simulink model "InterlockDeadtime3L"  (R2025b)
settings: Solver=FixedStepDiscrete  StartTime=0.0  StopTime=0.0000004  RelTol=1e-3
undefined symbols (not defined in the file): T_FPGA_clk
libraries: simulink x3, hdlsllib x3
settings Model: PacingRate=0.010000  Creator=info  LastModifiedBy=info
settings OptimizationCC: BlockReduction=off  ConditionallyExecuteInputs=off  DefaultParameterBehavior=Inlined
settings DebuggingCC: AlgebraicLoopMsg=error
settings HardwareCC: ProdBitPerPointer=32.0  ProdBitPerSizeT=32.0  ProdBitPerPtrDiffT=32.0  ProdLargestAtomicFloat=None  ProdIntDivRoundTo=Undefined  ProdEndianess=Unspecified  ProdWordSize=32.0  ProdHWDeviceType=ASIC/FPGA->ASIC/FPGA  TargetBitPerPointer=64.0  TargetBitPerSizeT=64.0  TargetBitPerPtrDiffT=64.0  TargetLongLongMode=on  TargetIntDivRoundTo=Zero  TargetEndianess=LittleEndian  TargetWordSize=64.0  TargetHWDeviceType=Custom Processor->MATLAB Host Computer  ProdEqTarget=off

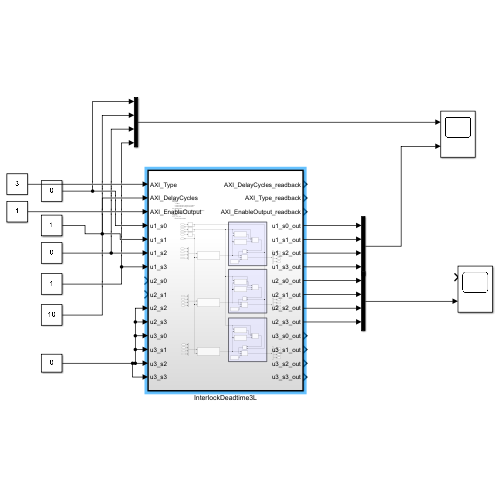
[thumbnail: Simulink's stored preview of the top-level diagram]
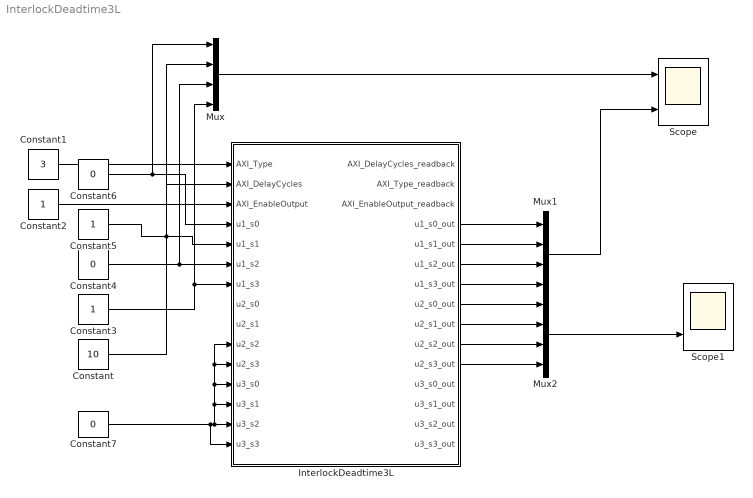
== system InterlockDeadtime3L ==
  Constant : Constant  Value=10  OutDataTypeStr=uint32  SampleTime=T_FPGA_clk
  Constant1 : Constant  Value=3  OutDataTypeStr=uint8  SampleTime=T_FPGA_clk
  Constant2 : Constant  OutDataTypeStr=boolean  SampleTime=T_FPGA_clk
  Constant3 : Constant  OutDataTypeStr=boolean  SampleTime=T_FPGA_clk
  Constant4 : Constant  Value=0  OutDataTypeStr=boolean  SampleTime=T_FPGA_clk
  Constant5 : Constant  OutDataTypeStr=boolean  SampleTime=T_FPGA_clk
  Constant6 : Constant  Value=0  OutDataTypeStr=boolean  SampleTime=T_FPGA_clk
  Constant7 : Constant  Value=0  OutDataTypeStr=boolean  SampleTime=T_FPGA_clk
  InterlockDeadtime3L : Subsystem  TreatAsAtomicUnit=on
  Mux : Mux
  Mux1 : Mux
  Mux2 : Mux
  Scope : Scope  NumInputPorts=2
      settings: ActiveDisplayYMinimum=-0.12499999999999997  ActiveDisplayYMaximum=1.125  DataLoggingVariableName=ScopeData2  DataLoggingSaveFormat=Array
  Scope1 : Scope  NumInputPorts=2
      settings: ActiveDisplayYMinimum=-0.12499999999999997  ActiveDisplayYMaximum=1.125  DataLoggingSaveFormat=Array
  wires:
  Constant/1 -> InterlockDeadtime3L/2(AXI_DelayCycles)
  Constant1/1 -> InterlockDeadtime3L/1(AXI_Type)
  Constant2/1 -> InterlockDeadtime3L/3(AXI_EnableOutput)
  Constant3/1 -> Mux/4, InterlockDeadtime3L/7(u1_s3)
  Constant6/1 -> Mux/1, InterlockDeadtime3L/4(u1_s0)
  Constant5/1 -> Mux/2, InterlockDeadtime3L/5(u1_s1)
  Constant4/1 -> Mux/3, InterlockDeadtime3L/6(u1_s2)
  Mux/1 -> Scope/1
  InterlockDeadtime3L/4(u1_s0_out) -> Mux1/1
  InterlockDeadtime3L/5(u1_s1_out) -> Mux1/2
  InterlockDeadtime3L/6(u1_s2_out) -> Mux1/3
  InterlockDeadtime3L/7(u1_s3_out) -> Mux1/4
  Mux1/1 -> Scope/2
  Constant7/1 -> InterlockDeadtime3L/15(u3_s3), InterlockDeadtime3L/14(u3_s2), InterlockDeadtime3L/13(u3_s1), InterlockDeadtime3L/12(u3_s0), InterlockDeadtime3L/11(u2_s3), InterlockDeadtime3L/10(u2_s2)
  InterlockDeadtime3L/8(u2_s0_out) -> Mux2/1
  InterlockDeadtime3L/10(u2_s2_out) -> Mux2/3
  InterlockDeadtime3L/9(u2_s1_out) -> Mux2/2
  InterlockDeadtime3L/11(u2_s3_out) -> Mux2/4
  Mux2/1 -> Scope1/2

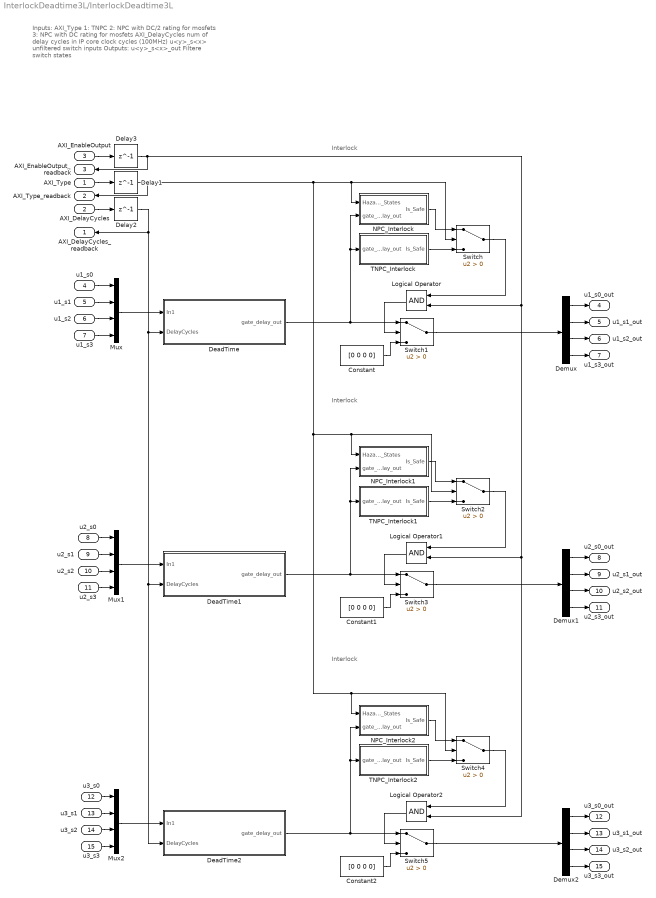
== system InterlockDeadtime3L/InterlockDeadtime3L ==
  note: Interlock
  note: Inputs:
      | AXI_Type
      | 1: TNPC
      | 2: NPC with DC/2 rating for mosfets
      | 3: NPC with DC rating for mosfets
      | AXI_DelayCycles
      | num of delay cycles in IP core clock cycles (100MHz)
      | u<y>_s<x>
      | unfiltered switch inputs
      | Outputs:
      | u<y>_s<x>_out
      | Filtere switch states
  note: Interlock
  note: Interlock
  AXI_Type : Inport
  AXI_DelayCycles : Inport  Port=2
  AXI_EnableOutput : Inport  Port=3
  u1_s0 : Inport  Port=4
  u1_s1 : Inport  Port=5
  u1_s2 : Inport  Port=6
  u1_s3 : Inport  Port=7
  u2_s0 : Inport  Port=8
  u2_s1 : Inport  Port=9
  u2_s2 : Inport  Port=10
  u2_s3 : Inport  Port=11
  u3_s0 : Inport  Port=12
  u3_s1 : Inport  Port=13
  u3_s2 : Inport  Port=14
  u3_s3 : Inport  Port=15
  Constant : Constant  Value=[0 0 0 0]  OutDataTypeStr=boolean
  Constant1 : Constant  Value=[0 0 0 0]  OutDataTypeStr=boolean
  Constant2 : Constant  Value=[0 0 0 0]  OutDataTypeStr=boolean
  DeadTime : Subsystem
  DeadTime1 : Subsystem
  DeadTime2 : Subsystem
  Delay1 : Delay  DelayLength=1
  Delay2 : Delay  DelayLength=1
  Delay3 : Delay  DelayLength=1
  Demux : Demux
  Demux1 : Demux
  Demux2 : Demux
  Logical Operator : Logic  AllPortsSameDT=off  OutDataTypeStr=boolean
  Logical Operator1 : Logic  AllPortsSameDT=off  OutDataTypeStr=boolean
  Logical Operator2 : Logic  AllPortsSameDT=off  OutDataTypeStr=boolean
  Mux : Mux
  Mux1 : Mux
  Mux2 : Mux
  NPC_Interlock : Subsystem
  NPC_Interlock1 : Subsystem
  NPC_Interlock2 : Subsystem
  Switch{,1..5} (6 alike) : Switch  Criteria=u2 > Threshold  SaturateOnIntegerOverflow=off  InputSameDT=off
  TNPC_Interlock : Subsystem
  TNPC_Interlock1 : Subsystem
  TNPC_Interlock2 : Subsystem
  AXI_DelayCycles_readback : Outport
  AXI_Type_readback : Outport  Port=2
  AXI_EnableOutput_readback : Outport  Port=3
  u1_s0_out : Outport  Port=4  OutDataTypeStr=boolean  VectorParamsAs1DForOutWhenUnconnected=off
  u1_s1_out : Outport  Port=5  OutDataTypeStr=boolean  VectorParamsAs1DForOutWhenUnconnected=off
  u1_s2_out : Outport  Port=6  OutDataTypeStr=boolean  VectorParamsAs1DForOutWhenUnconnected=off
  u1_s3_out : Outport  Port=7  OutDataTypeStr=boolean  VectorParamsAs1DForOutWhenUnconnected=off
  u2_s0_out : Outport  Port=8  OutDataTypeStr=boolean  VectorParamsAs1DForOutWhenUnconnected=off
  u2_s1_out : Outport  Port=9  OutDataTypeStr=boolean  VectorParamsAs1DForOutWhenUnconnected=off
  u2_s2_out : Outport  Port=10  OutDataTypeStr=boolean  VectorParamsAs1DForOutWhenUnconnected=off
  u2_s3_out : Outport  Port=11  OutDataTypeStr=boolean  VectorParamsAs1DForOutWhenUnconnected=off
  u3_s0_out : Outport  Port=12  OutDataTypeStr=boolean  VectorParamsAs1DForOutWhenUnconnected=off
  u3_s1_out : Outport  Port=13  OutDataTypeStr=boolean  VectorParamsAs1DForOutWhenUnconnected=off
  u3_s2_out : Outport  Port=14  OutDataTypeStr=boolean  VectorParamsAs1DForOutWhenUnconnected=off
  u3_s3_out : Outport  Port=15  OutDataTypeStr=boolean  VectorParamsAs1DForOutWhenUnconnected=off
  wires:
  u1_s0/1 -> Mux/1
  u1_s1/1 -> Mux/2
  u1_s2/1 -> Mux/3
  u1_s3/1 -> Mux/4
  Mux/1 -> DeadTime/1(In1)
  DeadTime/1(gate_delay_out) -> Switch1/1, NPC_Interlock/2(gate_delay_out), TNPC_Interlock/1(gate_delay_out)
  Demux/3 -> u1_s2_out/1
  Demux/4 -> u1_s3_out/1
  Demux/1 -> u1_s0_out/1
  Demux/2 -> u1_s1_out/1
  AXI_DelayCycles/1 -> Delay2/1
  AXI_Type/1 -> Delay1/1
  NPC_Interlock/1(Is_Safe) -> Switch/1
  TNPC_Interlock/1(Is_Safe) -> Switch/3
  Constant/1 -> Switch1/3
  Switch1/1 -> Demux/1
  Logical Operator/1 -> Switch1/2
  Switch/1 -> Logical Operator/1
  AXI_EnableOutput/1 -> Delay3/1
  Delay2/1 -> AXI_DelayCycles_readback/1, DeadTime2/2(DelayCycles), DeadTime1/2(DelayCycles), DeadTime/2(DelayCycles)
  Constant1/1 -> Switch3/3
  Switch3/1 -> Demux1/1
  Delay1/1 -> NPC_Interlock1/1(Hazard_States), Switch2/2, NPC_Interlock2/1(Hazard_States), Switch4/2, NPC_Interlock/1(Hazard_States), Switch/2, AXI_Type_readback/1
  TNPC_Interlock1/1(Is_Safe) -> Switch2/3
  Logical Operator1/1 -> Switch3/2
  NPC_Interlock1/1(Is_Safe) -> Switch2/1
  Switch2/1 -> Logical Operator1/1
  DeadTime1/1(gate_delay_out) -> Switch3/1, NPC_Interlock1/2(gate_delay_out), TNPC_Interlock1/1(gate_delay_out)
  Delay3/1 -> Logical Operator2/2, Logical Operator1/2, Logical Operator/2, AXI_EnableOutput_readback/1
  Constant2/1 -> Switch5/3
  Switch5/1 -> Demux2/1
  TNPC_Interlock2/1(Is_Safe) -> Switch4/3
  Logical Operator2/1 -> Switch5/2
  NPC_Interlock2/1(Is_Safe) -> Switch4/1
  Switch4/1 -> Logical Operator2/1
  DeadTime2/1(gate_delay_out) -> Switch5/1, NPC_Interlock2/2(gate_delay_out), TNPC_Interlock2/1(gate_delay_out)
  u2_s0/1 -> Mux1/1
  u2_s1/1 -> Mux1/2
  u2_s3/1 -> Mux1/4
  u2_s2/1 -> Mux1/3
  Mux1/1 -> DeadTime1/1(In1)
  u3_s0/1 -> Mux2/1
  u3_s1/1 -> Mux2/2
  u3_s2/1 -> Mux2/3
  u3_s3/1 -> Mux2/4
  Mux2/1 -> DeadTime2/1(In1)
  Demux1/4 -> u2_s3_out/1
  Demux1/1 -> u2_s0_out/1
  Demux1/2 -> u2_s1_out/1
  Demux1/3 -> u2_s2_out/1
  Demux2/4 -> u3_s3_out/1
  Demux2/1 -> u3_s0_out/1
  Demux2/2 -> u3_s1_out/1
  Demux2/3 -> u3_s2_out/1

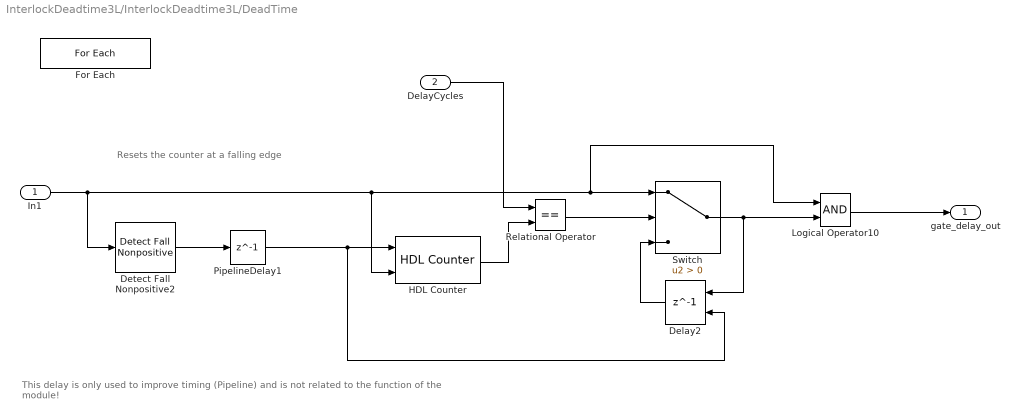
== system InterlockDeadtime3L/InterlockDeadtime3L/DeadTime ==
  note: This delay is only used to improve timing (Pipeline) and is not related to the function of the module!
  note: Resets the counter at a falling edge
  In1 : Inport  Partition=on  PartitionDimension=1  PartitionWidth=1  PartitionOffset=0
  DelayCycles : Inport  Port=2
  Delay2 : Delay  DelayLength=1  ExternalReset=Level  UseCircularBuffer=on
      settings: InputPortMap=u0,r5
  Detect Fall Nonpositive2 : simulink/Logic and Bit Operations/Detect Fall Nonpositive  vinit=0  OutDataTypeStr=boolean
  For Each : ForEach  DisableCoverage=on
  HDL Counter : hdlsllib/Sources/HDL Counter  CountType=Free running  CountInit=0  CountStep=1  CountMax=25  CountFromType=Initial value  CountFrom=0  CountResetPort=on  CountLoadPort=off  CountEnbPort=on  CountDirPort=off  CountHitOutputPort=off  CountDataType=Unsigned  CountWordLen=32  CountFracLen=0  CountSampTime=-1
  Logical Operator10 : Logic  AllPortsSameDT=off  OutDataTypeStr=boolean
  PipelineDelay1 : Delay  DelayLength=1
  Relational Operator : RelationalOperator  Operator===  OutDataTypeStr=boolean  RndMeth=Simplest  InputSameDT=off
  Switch : Switch  Criteria=u2 > Threshold  SaturateOnIntegerOverflow=off  InputSameDT=off
  gate_delay_out : Outport  ConcatenationDimension=1
  wires:
  Logical Operator10/1 -> gate_delay_out/1
  In1/1 -> Logical Operator10/1, Switch/1, HDL Counter/2, Detect Fall Nonpositive2/1
  HDL Counter/1 -> Relational Operator/2
  Delay2/1 -> Switch/3
  DelayCycles/1 -> Relational Operator/1
  Relational Operator/1 -> Switch/2
  PipelineDelay1/1 -> HDL Counter/1, Delay2/2
  Detect Fall Nonpositive2/1 -> PipelineDelay1/1
  Switch/1 -> Delay2/1, Logical Operator10/2

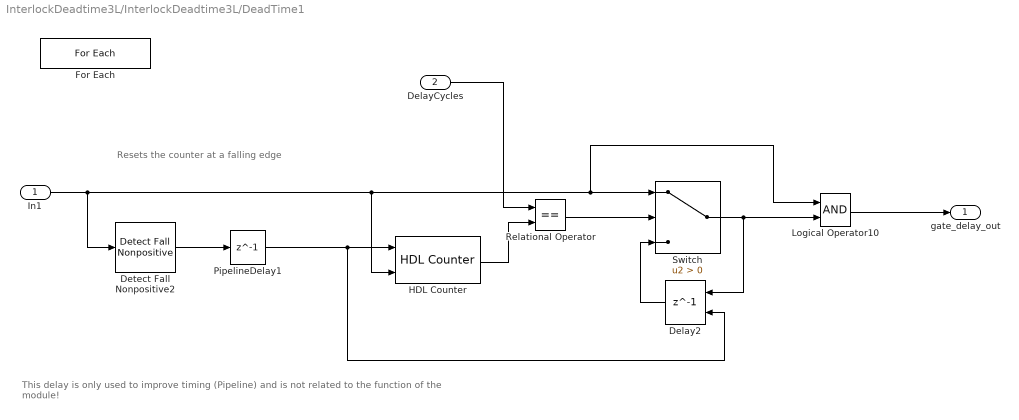
== system InterlockDeadtime3L/InterlockDeadtime3L/DeadTime1 ==
  note: This delay is only used to improve timing (Pipeline) and is not related to the function of the module!
  note: Resets the counter at a falling edge
  In1 : Inport  Partition=on  PartitionDimension=1  PartitionWidth=1  PartitionOffset=0
  DelayCycles : Inport  Port=2
  Delay2 : Delay  DelayLength=1  ExternalReset=Level  UseCircularBuffer=on
      settings: InputPortMap=u0,r5
  Detect Fall Nonpositive2 : simulink/Logic and Bit Operations/Detect Fall Nonpositive  vinit=0  OutDataTypeStr=boolean
  For Each : ForEach  DisableCoverage=on
  HDL Counter : hdlsllib/Sources/HDL Counter  CountType=Free running  CountInit=0  CountStep=1  CountMax=25  CountFromType=Initial value  CountFrom=0  CountResetPort=on  CountLoadPort=off  CountEnbPort=on  CountDirPort=off  CountHitOutputPort=off  CountDataType=Unsigned  CountWordLen=32  CountFracLen=0  CountSampTime=-1
  Logical Operator10 : Logic  AllPortsSameDT=off  OutDataTypeStr=boolean
  PipelineDelay1 : Delay  DelayLength=1
  Relational Operator : RelationalOperator  Operator===  OutDataTypeStr=boolean  RndMeth=Simplest  InputSameDT=off
  Switch : Switch  Criteria=u2 > Threshold  SaturateOnIntegerOverflow=off  InputSameDT=off
  gate_delay_out : Outport  ConcatenationDimension=1
  wires:
  Logical Operator10/1 -> gate_delay_out/1
  In1/1 -> Logical Operator10/1, Switch/1, HDL Counter/2, Detect Fall Nonpositive2/1
  HDL Counter/1 -> Relational Operator/2
  Delay2/1 -> Switch/3
  DelayCycles/1 -> Relational Operator/1
  Relational Operator/1 -> Switch/2
  PipelineDelay1/1 -> HDL Counter/1, Delay2/2
  Detect Fall Nonpositive2/1 -> PipelineDelay1/1
  Switch/1 -> Delay2/1, Logical Operator10/2

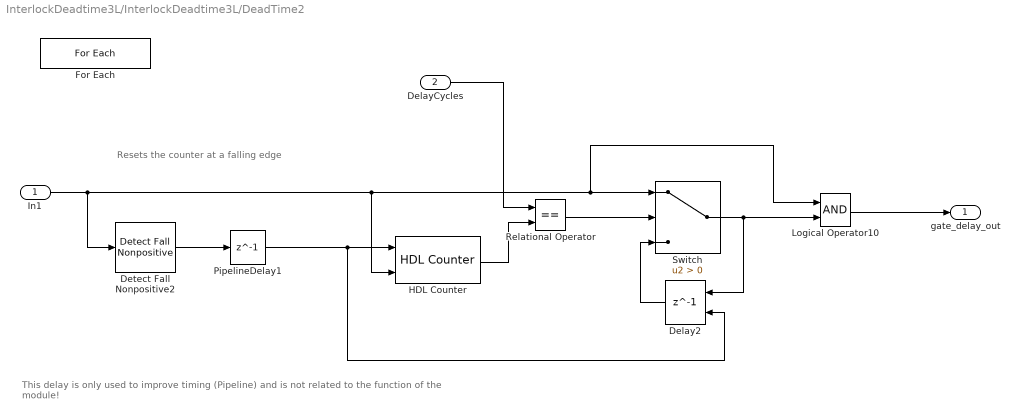
== system InterlockDeadtime3L/InterlockDeadtime3L/DeadTime2 ==
  note: This delay is only used to improve timing (Pipeline) and is not related to the function of the module!
  note: Resets the counter at a falling edge
  In1 : Inport  Partition=on  PartitionDimension=1  PartitionWidth=1  PartitionOffset=0
  DelayCycles : Inport  Port=2
  Delay2 : Delay  DelayLength=1  ExternalReset=Level  UseCircularBuffer=on
      settings: InputPortMap=u0,r5
  Detect Fall Nonpositive2 : simulink/Logic and Bit Operations/Detect Fall Nonpositive  vinit=0  OutDataTypeStr=boolean
  For Each : ForEach  DisableCoverage=on
  HDL Counter : hdlsllib/Sources/HDL Counter  CountType=Free running  CountInit=0  CountStep=1  CountMax=25  CountFromType=Initial value  CountFrom=0  CountResetPort=on  CountLoadPort=off  CountEnbPort=on  CountDirPort=off  CountHitOutputPort=off  CountDataType=Unsigned  CountWordLen=32  CountFracLen=0  CountSampTime=-1
  Logical Operator10 : Logic  AllPortsSameDT=off  OutDataTypeStr=boolean
  PipelineDelay1 : Delay  DelayLength=1
  Relational Operator : RelationalOperator  Operator===  OutDataTypeStr=boolean  RndMeth=Simplest  InputSameDT=off
  Switch : Switch  Criteria=u2 > Threshold  SaturateOnIntegerOverflow=off  InputSameDT=off
  gate_delay_out : Outport  ConcatenationDimension=1
  wires:
  Logical Operator10/1 -> gate_delay_out/1
  In1/1 -> Logical Operator10/1, Switch/1, HDL Counter/2, Detect Fall Nonpositive2/1
  HDL Counter/1 -> Relational Operator/2
  Delay2/1 -> Switch/3
  DelayCycles/1 -> Relational Operator/1
  Relational Operator/1 -> Switch/2
  PipelineDelay1/1 -> HDL Counter/1, Delay2/2
  Detect Fall Nonpositive2/1 -> PipelineDelay1/1
  Switch/1 -> Delay2/1, Logical Operator10/2

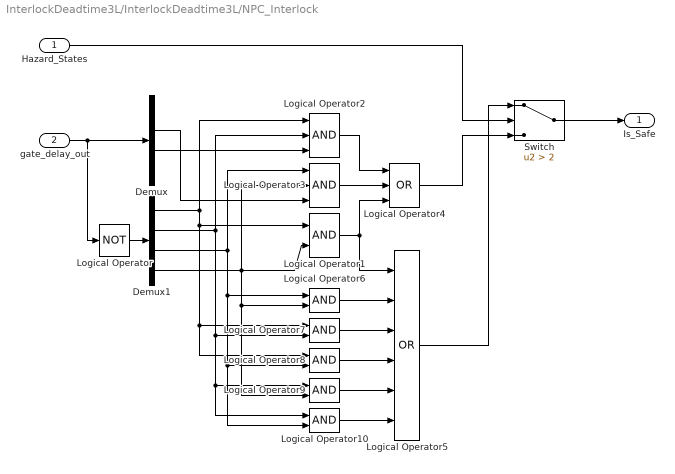
== system InterlockDeadtime3L/InterlockDeadtime3L/NPC_Interlock ==
  Hazard_States : Inport
  gate_delay_out : Inport  Port=2
  Demux : Demux
  Demux1 : Demux
  Logical Operator : Logic  Operator=NOT  AllPortsSameDT=off  OutDataTypeStr=boolean
  Logical Operator{1,6..10} (6 alike) : Logic  AllPortsSameDT=off  OutDataTypeStr=boolean
  Logical Operator2 : Logic  Inputs=3  AllPortsSameDT=off  OutDataTypeStr=boolean
  Logical Operator3 : Logic  Inputs=3  AllPortsSameDT=off  OutDataTypeStr=boolean
  Logical Operator4 : Logic  Operator=OR  Inputs=3  AllPortsSameDT=off  OutDataTypeStr=boolean
  Logical Operator5 : Logic  Operator=OR  Inputs=6  AllPortsSameDT=off  OutDataTypeStr=boolean
  Switch : Switch  Criteria=u2 > Threshold  Threshold=2  SaturateOnIntegerOverflow=off  InputSameDT=off
  Is_Safe : Outport
  wires:
  gate_delay_out/1 -> Logical Operator/1, Demux/1
  Logical Operator/1 -> Demux1/1
  Demux1/1 -> Logical Operator7/1, Logical Operator8/1, Logical Operator1/1, Logical Operator2/1
  Demux1/4 -> Logical Operator9/2, Logical Operator6/2, Logical Operator1/2, Logical Operator3/2
  Demux1/2 -> Logical Operator2/2, Logical Operator10/1, Logical Operator9/1, Logical Operator7/2
  Demux/3 -> Logical Operator2/3
  Demux/2 -> Logical Operator3/3
  Demux1/3 -> Logical Operator6/1, Logical Operator10/2, Logical Operator8/2, Logical Operator3/1
  Logical Operator2/1 -> Logical Operator4/1
  Logical Operator1/1 -> Logical Operator5/1, Logical Operator4/3
  Logical Operator3/1 -> Logical Operator4/2
  Switch/1 -> Is_Safe/1
  Hazard_States/1 -> Switch/2
  Logical Operator4/1 -> Switch/3
  Logical Operator10/1 -> Logical Operator5/6
  Logical Operator9/1 -> Logical Operator5/5
  Logical Operator8/1 -> Logical Operator5/4
  Logical Operator7/1 -> Logical Operator5/3
  Logical Operator6/1 -> Logical Operator5/2
  Logical Operator5/1 -> Switch/1

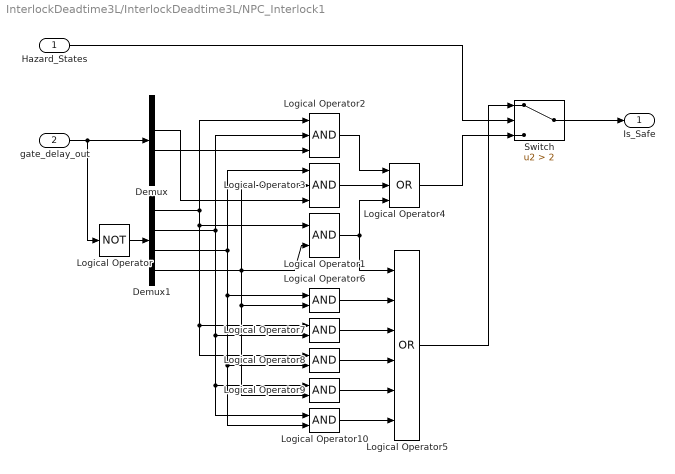
== system InterlockDeadtime3L/InterlockDeadtime3L/NPC_Interlock1 ==
  Hazard_States : Inport
  gate_delay_out : Inport  Port=2
  Demux : Demux
  Demux1 : Demux
  Logical Operator : Logic  Operator=NOT  AllPortsSameDT=off  OutDataTypeStr=boolean
  Logical Operator{1,6..10} (6 alike) : Logic  AllPortsSameDT=off  OutDataTypeStr=boolean
  Logical Operator2 : Logic  Inputs=3  AllPortsSameDT=off  OutDataTypeStr=boolean
  Logical Operator3 : Logic  Inputs=3  AllPortsSameDT=off  OutDataTypeStr=boolean
  Logical Operator4 : Logic  Operator=OR  Inputs=3  AllPortsSameDT=off  OutDataTypeStr=boolean
  Logical Operator5 : Logic  Operator=OR  Inputs=6  AllPortsSameDT=off  OutDataTypeStr=boolean
  Switch : Switch  Criteria=u2 > Threshold  Threshold=2  SaturateOnIntegerOverflow=off  InputSameDT=off
  Is_Safe : Outport
  wires:
  gate_delay_out/1 -> Logical Operator/1, Demux/1
  Logical Operator/1 -> Demux1/1
  Demux1/1 -> Logical Operator7/1, Logical Operator8/1, Logical Operator1/1, Logical Operator2/1
  Demux1/4 -> Logical Operator9/2, Logical Operator6/2, Logical Operator1/2, Logical Operator3/2
  Demux1/2 -> Logical Operator2/2, Logical Operator10/1, Logical Operator9/1, Logical Operator7/2
  Demux/3 -> Logical Operator2/3
  Demux/2 -> Logical Operator3/3
  Demux1/3 -> Logical Operator6/1, Logical Operator10/2, Logical Operator8/2, Logical Operator3/1
  Logical Operator2/1 -> Logical Operator4/1
  Logical Operator1/1 -> Logical Operator5/1, Logical Operator4/3
  Logical Operator3/1 -> Logical Operator4/2
  Switch/1 -> Is_Safe/1
  Hazard_States/1 -> Switch/2
  Logical Operator4/1 -> Switch/3
  Logical Operator10/1 -> Logical Operator5/6
  Logical Operator9/1 -> Logical Operator5/5
  Logical Operator8/1 -> Logical Operator5/4
  Logical Operator7/1 -> Logical Operator5/3
  Logical Operator6/1 -> Logical Operator5/2
  Logical Operator5/1 -> Switch/1

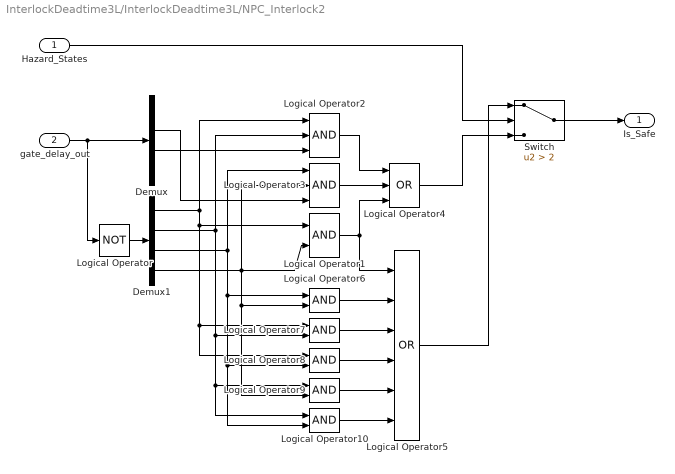
== system InterlockDeadtime3L/InterlockDeadtime3L/NPC_Interlock2 ==
  Hazard_States : Inport
  gate_delay_out : Inport  Port=2
  Demux : Demux
  Demux1 : Demux
  Logical Operator : Logic  Operator=NOT  AllPortsSameDT=off  OutDataTypeStr=boolean
  Logical Operator{1,6..10} (6 alike) : Logic  AllPortsSameDT=off  OutDataTypeStr=boolean
  Logical Operator2 : Logic  Inputs=3  AllPortsSameDT=off  OutDataTypeStr=boolean
  Logical Operator3 : Logic  Inputs=3  AllPortsSameDT=off  OutDataTypeStr=boolean
  Logical Operator4 : Logic  Operator=OR  Inputs=3  AllPortsSameDT=off  OutDataTypeStr=boolean
  Logical Operator5 : Logic  Operator=OR  Inputs=6  AllPortsSameDT=off  OutDataTypeStr=boolean
  Switch : Switch  Criteria=u2 > Threshold  Threshold=2  SaturateOnIntegerOverflow=off  InputSameDT=off
  Is_Safe : Outport
  wires:
  gate_delay_out/1 -> Logical Operator/1, Demux/1
  Logical Operator/1 -> Demux1/1
  Demux1/1 -> Logical Operator7/1, Logical Operator8/1, Logical Operator1/1, Logical Operator2/1
  Demux1/4 -> Logical Operator9/2, Logical Operator6/2, Logical Operator1/2, Logical Operator3/2
  Demux1/2 -> Logical Operator2/2, Logical Operator10/1, Logical Operator9/1, Logical Operator7/2
  Demux/3 -> Logical Operator2/3
  Demux/2 -> Logical Operator3/3
  Demux1/3 -> Logical Operator6/1, Logical Operator10/2, Logical Operator8/2, Logical Operator3/1
  Logical Operator2/1 -> Logical Operator4/1
  Logical Operator1/1 -> Logical Operator5/1, Logical Operator4/3
  Logical Operator3/1 -> Logical Operator4/2
  Switch/1 -> Is_Safe/1
  Hazard_States/1 -> Switch/2
  Logical Operator4/1 -> Switch/3
  Logical Operator10/1 -> Logical Operator5/6
  Logical Operator9/1 -> Logical Operator5/5
  Logical Operator8/1 -> Logical Operator5/4
  Logical Operator7/1 -> Logical Operator5/3
  Logical Operator6/1 -> Logical Operator5/2
  Logical Operator5/1 -> Switch/1

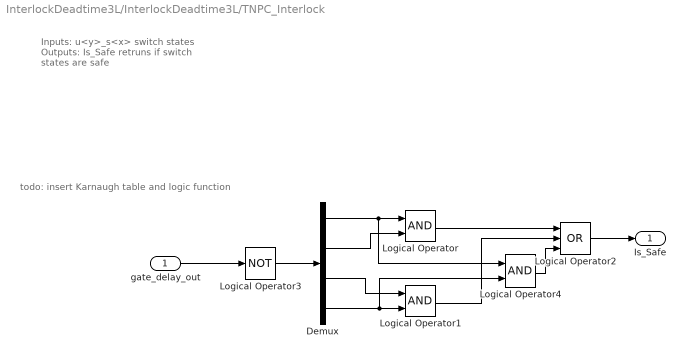
== system InterlockDeadtime3L/InterlockDeadtime3L/TNPC_Interlock ==
  note: todo: insert Karnaugh table and logic function
  note: Inputs:
      | u<y>_s<x>
      | switch states
      | Outputs:
      | Is_Safe
      | retruns if switch states are safe
  gate_delay_out : Inport
  Demux : Demux
  Logical Operator : Logic  AllPortsSameDT=off  OutDataTypeStr=boolean
  Logical Operator1 : Logic  AllPortsSameDT=off  OutDataTypeStr=boolean
  Logical Operator2 : Logic  Operator=OR  Inputs=3  AllPortsSameDT=off  OutDataTypeStr=boolean
  Logical Operator3 : Logic  Operator=NOT  AllPortsSameDT=off  OutDataTypeStr=boolean
  Logical Operator4 : Logic  AllPortsSameDT=off  OutDataTypeStr=boolean
  Is_Safe : Outport
  wires:
  gate_delay_out/1 -> Logical Operator3/1
  Demux/1 -> Logical Operator4/1, Logical Operator/1
  Demux/2 -> Logical Operator/2
  Demux/4 -> Logical Operator4/2, Logical Operator1/2
  Demux/3 -> Logical Operator1/1
  Logical Operator1/1 -> Logical Operator2/2
  Logical Operator/1 -> Logical Operator2/1
  Logical Operator3/1 -> Demux/1
  Logical Operator4/1 -> Logical Operator2/3
  Logical Operator2/1 -> Is_Safe/1

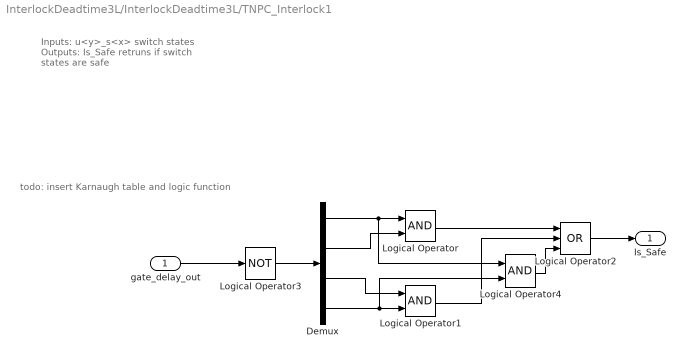
== system InterlockDeadtime3L/InterlockDeadtime3L/TNPC_Interlock1 ==
  note: todo: insert Karnaugh table and logic function
  note: Inputs:
      | u<y>_s<x>
      | switch states
      | Outputs:
      | Is_Safe
      | retruns if switch states are safe
  gate_delay_out : Inport
  Demux : Demux
  Logical Operator : Logic  AllPortsSameDT=off  OutDataTypeStr=boolean
  Logical Operator1 : Logic  AllPortsSameDT=off  OutDataTypeStr=boolean
  Logical Operator2 : Logic  Operator=OR  Inputs=3  AllPortsSameDT=off  OutDataTypeStr=boolean
  Logical Operator3 : Logic  Operator=NOT  AllPortsSameDT=off  OutDataTypeStr=boolean
  Logical Operator4 : Logic  AllPortsSameDT=off  OutDataTypeStr=boolean
  Is_Safe : Outport
  wires:
  gate_delay_out/1 -> Logical Operator3/1
  Demux/1 -> Logical Operator4/1, Logical Operator/1
  Demux/2 -> Logical Operator/2
  Demux/4 -> Logical Operator4/2, Logical Operator1/2
  Demux/3 -> Logical Operator1/1
  Logical Operator1/1 -> Logical Operator2/2
  Logical Operator/1 -> Logical Operator2/1
  Logical Operator3/1 -> Demux/1
  Logical Operator4/1 -> Logical Operator2/3
  Logical Operator2/1 -> Is_Safe/1

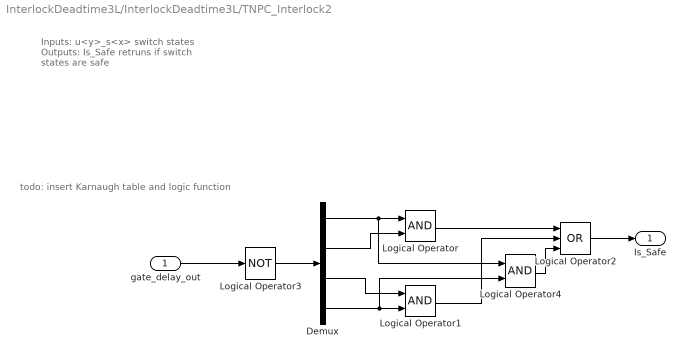
== system InterlockDeadtime3L/InterlockDeadtime3L/TNPC_Interlock2 ==
  note: todo: insert Karnaugh table and logic function
  note: Inputs:
      | u<y>_s<x>
      | switch states
      | Outputs:
      | Is_Safe
      | retruns if switch states are safe
  gate_delay_out : Inport
  Demux : Demux
  Logical Operator : Logic  AllPortsSameDT=off  OutDataTypeStr=boolean
  Logical Operator1 : Logic  AllPortsSameDT=off  OutDataTypeStr=boolean
  Logical Operator2 : Logic  Operator=OR  Inputs=3  AllPortsSameDT=off  OutDataTypeStr=boolean
  Logical Operator3 : Logic  Operator=NOT  AllPortsSameDT=off  OutDataTypeStr=boolean
  Logical Operator4 : Logic  AllPortsSameDT=off  OutDataTypeStr=boolean
  Is_Safe : Outport
  wires:
  gate_delay_out/1 -> Logical Operator3/1
  Demux/1 -> Logical Operator4/1, Logical Operator/1
  Demux/2 -> Logical Operator/2
  Demux/4 -> Logical Operator4/2, Logical Operator1/2
  Demux/3 -> Logical Operator1/1
  Logical Operator1/1 -> Logical Operator2/2
  Logical Operator/1 -> Logical Operator2/1
  Logical Operator3/1 -> Demux/1
  Logical Operator4/1 -> Logical Operator2/3
  Logical Operator2/1 -> Is_Safe/1
